simulink model "main_train_proto_discrete"  (Simulink 7.8)
settings: Solver=ode45  StartTime=0.0  StopTime=5  RelTol=1e-3
settings Model: Creator=imac  LastModifiedBy=aitor
settings DebuggingCC: FcnCallInpInsideContextMsg=Use local settings

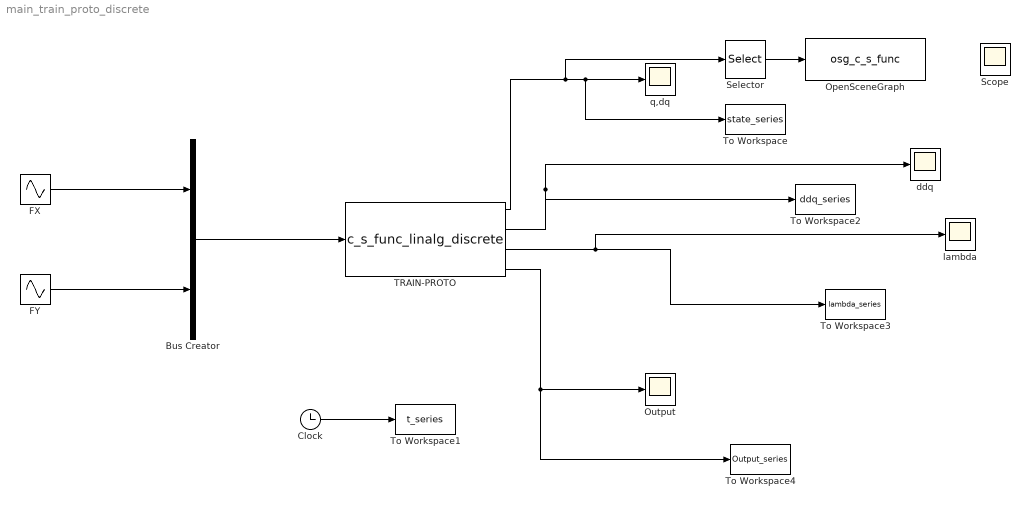
== system main_train_proto_discrete ==
  Bus Creator : BusCreator  Inputs=2
  Clock : Clock
  FX : Sin  Description=FX  Frequency=0  Phase=pi/2  SampleTime=0
  FY : Sin  Amplitude=2  Frequency=0  Phase=pi/2  SampleTime=0
  OpenSceneGraph : S-Function  FunctionName=osg_c_s_func  EnableBusSupport=off
  Output : Scope
      settings: YMin=-7000  YMax=7000  SaveName=ScopeData3  SampleInput=on  SampleTime=0.01
  Scope : Scope
      settings: SaveName=ScopeData4
  Selector : Selector  InputPortWidth=12  IndexOptions=Index vector (dialog)  Indices=[1 2 3 4 5 6]  OutputSizes=1
  TRAIN-PROTO : S-Function  FunctionName=c_s_func_linalg_discrete  Parameters=q dq param Delta_t  EnableBusSupport=off
      mask Type: S-function: mycsfunc
      mask Description: This is a S-function that does the continuous state space system.
      mask Display: disp('[M , Phi_q''] [ddq]\n[Phi_q , 0] [lambda]\n=\n [Q ] \n   [gamma] ');
  To Workspace : ToWorkspace  VariableName=state_series  SampleTime=0.01  SaveFormat=Array
  To Workspace1 : ToWorkspace  VariableName=t_series  SampleTime=0.01  SaveFormat=Array
  To Workspace2 : ToWorkspace  VariableName=ddq_series  SampleTime=0.01  SaveFormat=Array
  To Workspace3 : ToWorkspace  VariableName=lambda_series  SampleTime=0.01  SaveFormat=Array
  To Workspace4 : ToWorkspace  VariableName=Output_series  SampleTime=0.01  SaveFormat=Array
  ddq : Scope
      settings: YMin=-0.05  YMax=0.6  SampleInput=on  SampleTime=0.01
  lambda : Scope
      settings: TimeRange=5  YMin=-2250  YMax=1750  SaveName=ScopeData2  SampleInput=on  SampleTime=0.01
  q,dq : Scope
      settings: YMin=-0.45  YMax=0.45  SampleInput=on  SampleTime=0.01
  wires:
  Clock/1 -> To Workspace1/1
  TRAIN-PROTO/1 -> q,dq/1, To Workspace/1, Selector/1
  TRAIN-PROTO/2 -> ddq/1, To Workspace2/1
  TRAIN-PROTO/3 -> lambda/1, To Workspace3/1
  TRAIN-PROTO/4 -> Output/1, To Workspace4/1
  Selector/1 -> OpenSceneGraph/1
  ? -> Scope/1
  Bus Creator/1 -> TRAIN-PROTO/1
  FX/1 -> Bus Creator/1
  FY/1 -> Bus Creator/2
